simulink model "abslut50_fixpt16"  (R2021b)
settings: Solver=VariableStepAuto  StartTime=0.0  StopTime=99  RelTol=1e-3
undefined symbols (not defined in the file): figd2104, xcu250
libraries: hdlBasic x391, vmcUtilities x1
(part 4 of 4)

== matlab function abslut50_fixpt16/MATLAB Function ==
  data: in input; out output; exact input
%function y = fcn(u,x)
%y = immse(u,x);
function out = mse_f(in,exact)
    out = (in - exact).^2;
end

== matlab function abslut50_fixpt16/MATLAB Function2 ==
  data: x input; out output; y input
function out = fcn(x,y)
out = sqrt(x.^2 + y.^2);
